simulink model "generar_signal"  (R2014a)
settings: Solver=ode45  StartTime=0.0  StopTime=1  RelTol=1e-3
settings Model: Creator=Wels  LastModifiedBy=Wels

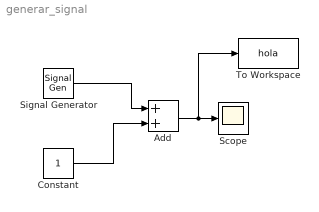
== system generar_signal ==
  Add : Sum
  Constant : Constant
  Scope : Scope
      settings: YMin=0.95  YMax=1.05
  Signal Generator : SignalGenerator  Amplitude=0.5  Frequency=60
  To Workspace : ToWorkspace  VariableName=hola  SampleTime=0.001
  wires:
  Constant/1 -> Add/2
  Signal Generator/1 -> Add/1
  Add/1 -> To Workspace/1, Scope/1
